simulink model "submultiplier"  (R2018b)
settings: Solver=VariableStepAuto  StartTime=0.0  StopTime=10.0  RelTol=1e-3
settings Model: Creator=annat  LastModifiedBy=annat

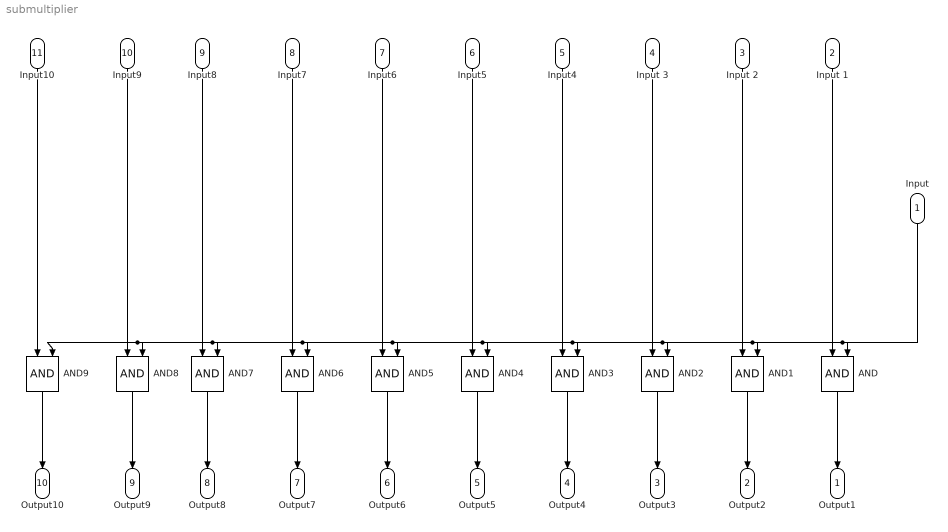
== system submultiplier ==
  Input : Inport
  Input 1 : Inport  Port=2
  Input 2 : Inport  Port=3
  Input 3 : Inport  Port=4
  Input4 : Inport  Port=5
  Input5 : Inport  Port=6
  Input6 : Inport  Port=7
  Input7 : Inport  Port=8
  Input8 : Inport  Port=9
  Input9 : Inport  Port=10
  Input10 : Inport  Port=11
  AND{,1..9} (10 alike) : Logic  IconShape=distinctive  AllPortsSameDT=off  OutDataTypeStr=boolean
  Output1 : Outport
  Output2 : Outport  Port=2
  Output3 : Outport  Port=3
  Output4 : Outport  Port=4
  Output5 : Outport  Port=5
  Output6 : Outport  Port=6
  Output7 : Outport  Port=7
  Output8 : Outport  Port=8
  Output9 : Outport  Port=9
  Output10 : Outport  Port=10
  wires:
  AND/1 -> Output1/1
  AND1/1 -> Output2/1
  AND3/1 -> Output4/1
  AND2/1 -> Output3/1
  AND6/1 -> Output7/1
  AND7/1 -> Output8/1
  AND5/1 -> Output6/1
  AND4/1 -> Output5/1
  Input5/1 -> AND4/1
  Input 3/1 -> AND2/1
  Input 2/1 -> AND1/1
  Input7/1 -> AND6/1
  Input4/1 -> AND3/1
  Input 1/1 -> AND/1
  Input6/1 -> AND5/1
  Input8/1 -> AND7/1
  Input10/1 -> AND9/1
  AND9/1 -> Output10/1
  Input/1 -> AND9/2, AND8/2, AND7/2, AND6/2, AND5/2, AND4/2, AND3/2, AND2/2, AND1/2, AND/2
  AND8/1 -> Output9/1
  Input9/1 -> AND8/1
